simulink model "sRes_nt"  (R2018b)
settings: Solver=ode23tb  StartTime=0.0  StopTime=7  MaxStep=10e-6  RelTol=1e-4  EnableMultiTasking=on
libraries: powerlib x49
settings Model: SimulationMode=accelerator  Creator=Gong Linxiao  LastModifiedBy=vibra
settings DataIOCC: LimitDataPoints=on  SaveFormat=Array
settings OptimizationCC: LifeSpan=inf
settings DebuggingCC: SolverPrmCheckMsg=warning  SFUnexpectedBacktrackingDiag=warning  SFNoUnconditionalDefaultTransitionDiag=warning  SFExecutionAtInitializationDiag=none
settings HardwareCC: ProdBitPerPointer=32  ProdBitPerSizeT=32  ProdBitPerPtrDiffT=32  ProdLargestAtomicFloat=None  ProdIntDivRoundTo=Undefined  ProdEndianess=Unspecified  ProdWordSize=32  ProdHWDeviceType=32-bit Generic
settings ModelReferenceCC: PropagateSignalLabelsOutOfModel=off
settings SFSimCC: SimUseLocalCustomCode=off
settings RTWCC: RTWUseLocalCustomCode=off
settings CodeAppCC: StateflowObjectComments=on
settings GRTTargetCC: TargetLangStandard=C89/C90 (ANSI)  GeneratePreprocessorConditionals=Disable all
settings ConfigComp: CovMetricSettings=dw  CovHtmlReporting=on  CovSaveCumulativeToWorkspaceVar=on  CovSaveSingleToWorkspaceVar=on  CovExternalEMLEnable=off  CovSFcnEnable=off
settings SimscapeCC: SimscapeNormalizeSystem=off

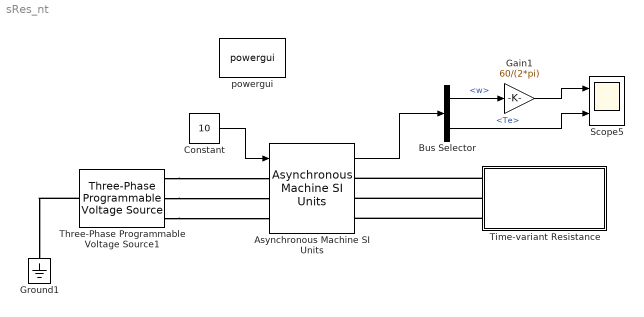
== system sRes_nt ==
  Asynchronous Machine SI Units : powerlib/Machines/Asynchronous Machine SI Units  RotorType=Wound  PresetModel="15:  5.4 HP (4KW)   400 V  50Hz 1430 RPM"  MechanicalLoad=Torque Tm  ShowDetailedParameters=on  ReferenceFrame=Stationary  Units=SI  MeasurementBus=on  NominalParameters=[4000 400 50]  Stator=[1.405 0.005839]  Rotor=[1.395 0.005839]  Cage1=[ 0.022 0.226/377]  Cage2=[ 0.022 0.226/377]  Lm=0.1722  Mechanical=[0.0131 0.002985 2]  PolePairs=2  InitialConditions=[1 0 0 0 0 0 0 0]  SimulateSaturation=off  Saturation=[14.03593122, 27.81365428, 53.79336849, 72.68890987, 97.98006896, 148.6815601, 215.7428561, 302.9841135, 420.4778367 ; 230, 322, 414, 460, 506, 552, 598, 644, 690]  LoadFlowParameters=1492000  TsPowergui=0  TsBlock=-1  IterativeModel=Trapezoidal non iterative  IterativeDiscreteModel=Trapezoidal non iterative  Pmec=0
      settings: SourceProductName=Simscape Electrical
  Bus Selector : BusSelector  OutputSignals=w,Te
  Constant : Constant  Value=10  SampleTime=Inf
  Gain1 : Gain  Gain=60/(2*pi)
  Ground1 : powerlib/Elements/Ground  LConnTagsString=a
      settings: SourceProductName=Simscape Electrical
  Scope5 : Scope  NumInputPorts=2
  Three-Phase Programmable Voltage Source1 : powerlib/Electrical Sources/Three-Phase Programmable Voltage Source  PositiveSequence="[400  0 50]"  VariationEntity=None  VariationType=Table of time-amplitude pairs  VariationTypeAlt=Step  VariationStep=20  VariationRate=30  VariationMagnitude=0.3  VariationFrequency=2  VariationTiming=[1 5]  VariationPhaseA=off  Amplitudes=[1 0.8 1.2 1.0]  TimeValues=[0 0.1 0.15 0.2]  HarmonicGeneration=off  HarmonicA=[3 0.2 -25 0]  HarmonicB=[2 0.15 35 2]  Timing="[0.05  3]"  BusType=PV  Pref=0  Qref=0  Qmin=-inf  Qmax=inf
      settings: SourceProductName=Simscape Electrical
  Time-variant Resistance : Subsystem
  powergui : powerlib/powergui  Priority=1  SimulationMode=Continuous  SampleTime=50e-6  frequency=60  Iterations=50  frequencyindice=50  Pbase=100e6  ErrMax=1e-4  UnitsV=kV  UnitsW=MW  buscounter=0  FunctionMessages=off  echomessages=off  EnableUseOfTLC=off  CurrentSourceSwitches=on  DisableSnubberDevices=off  DisableRonSwitches=off  DisableVfSwitches=off  DisplayEquations=off  SolverType=Tustin  Interpol=off  ExternalGateDelay=off  methode=off  Ts=0  x0status=steady  SPID=off  SwTol=0  HookPort=off  RestoreLinks=warning  ResistiveCurrentMeasurement=off  Frange=[0:2:500]  Ylog=off  Xlog=on  ShowGrid=off  save=off  variable=ZData  structure=0  ZoomFFT=off  StartTime=0.0  cycles=1  DisplayStyle=1  fundamental=60  FreqAxis=off  MaxFrequency=1000  frequencyindicesteady=1  RmsSteady=2  display=off
  wires:
  Constant/1 -> Asynchronous Machine SI Units/1
  Asynchronous Machine SI Units/1 -> Bus Selector/1
  Bus Selector/1 -> Gain1/1  "<w>"
  Gain1/1 -> Scope5/1
  Bus Selector/2 -> Scope5/2  "<Te>"
  connections:
  Three-Phase Programmable Voltage Source1/LConn1 -- Ground1/LConn1
  Three-Phase Programmable Voltage Source1/RConn1 -- Asynchronous Machine SI Units/LConn1
  Three-Phase Programmable Voltage Source1/RConn2 -- Asynchronous Machine SI Units/LConn2
  Three-Phase Programmable Voltage Source1/RConn3 -- Asynchronous Machine SI Units/LConn3
  Time-variant Resistance/LConn1 -- Asynchronous Machine SI Units/RConn1
  Time-variant Resistance/LConn2 -- Asynchronous Machine SI Units/RConn2
  Time-variant Resistance/LConn3 -- Asynchronous Machine SI Units/RConn3

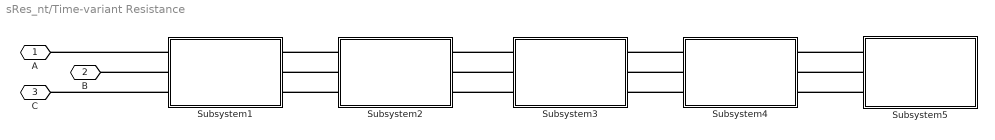
== system sRes_nt/Time-variant Resistance ==
  Subsystem1 : Subsystem
  Subsystem2 : Subsystem
  Subsystem3 : Subsystem
  Subsystem4 : Subsystem
  Subsystem5 : Subsystem
  A : PMIOPort  Side=Left
  B : PMIOPort  Port=2  Side=Left
  C : PMIOPort  Port=3  Side=Left
  connections:
  Subsystem3/LConn3 -- Subsystem2/RConn3
  Subsystem2/LConn2 -- Subsystem1/RConn2
  Subsystem3/LConn2 -- Subsystem2/RConn2
  Subsystem2/LConn3 -- Subsystem1/RConn3
  Subsystem1/LConn3 -- C/RConn1
  Subsystem4/LConn3 -- Subsystem3/RConn3
  Subsystem5/LConn2 -- Subsystem4/RConn2
  Subsystem4/LConn2 -- Subsystem3/RConn2
  Subsystem3/LConn1 -- Subsystem2/RConn1
  Subsystem4/LConn1 -- Subsystem3/RConn1
  Subsystem5/LConn1 -- Subsystem4/RConn1
  Subsystem2/LConn1 -- Subsystem1/RConn1
  Subsystem5/LConn3 -- Subsystem4/RConn3
  Subsystem1/LConn2 -- B/RConn1
  Subsystem1/LConn1 -- A/RConn1

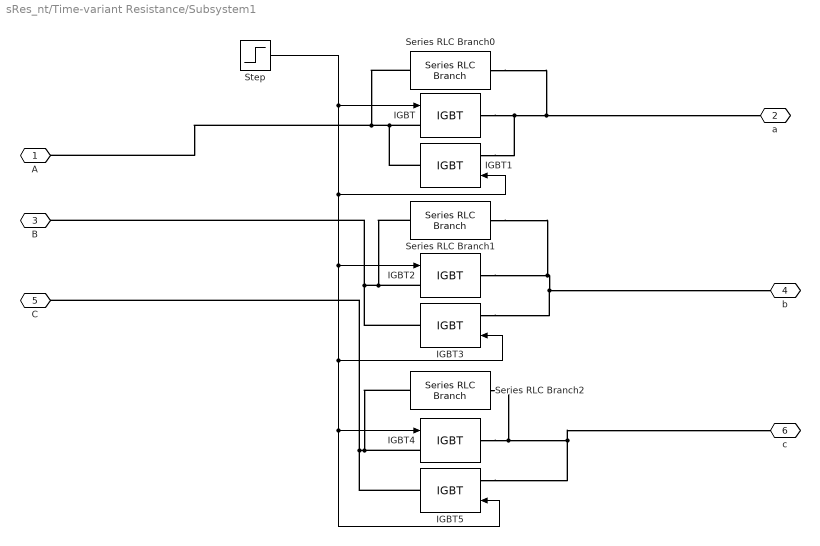
== system sRes_nt/Time-variant Resistance/Subsystem1 ==
  IGBT{,1..5} (6 alike) : powerlib/Power Electronics/IGBT  Ron=1e-5  Lon=0  Vf=0  Tf=1e-6  Tt=2e-6  IC=0  Rs=inf  Cs=inf  Measurements=off
  Series RLC Branch0 : powerlib/Elements/Series RLC Branch  LConnTagsString=__new0  RConnTagsString=__new0  BranchType=R  Resistance=1  Inductance=1e-3  SetiL0=off  InitialCurrent=0  Capacitance=1e-6  Setx0=off  InitialVoltage=0  Measurements=None
  Series RLC Branch1 : powerlib/Elements/Series RLC Branch  LConnTagsString=__new0  RConnTagsString=__new0  BranchType=R  Resistance=1  Inductance=1e-3  SetiL0=off  InitialCurrent=0  Capacitance=1e-6  Setx0=off  InitialVoltage=0  Measurements=None
  Series RLC Branch2 : powerlib/Elements/Series RLC Branch  LConnTagsString=__new0  RConnTagsString=__new0  BranchType=R  Resistance=1  Inductance=1e-3  SetiL0=off  InitialCurrent=0  Capacitance=1e-6  Setx0=off  InitialVoltage=0  Measurements=None
  Step : Step  Before=1  After=0  SampleTime=0
  A : PMIOPort  Side=Left
  a : PMIOPort  Port=2  Side=Right
  B : PMIOPort  Port=3  Side=Left
  b : PMIOPort  Port=4  Side=Right
  C : PMIOPort  Port=5  Side=Left
  c : PMIOPort  Port=6  Side=Right
  wires:
  Step/1 -> IGBT2/1, IGBT5/1, IGBT4/1, IGBT3/1, IGBT1/1, IGBT/1
  connections:
  IGBT2/RConn1 -- Series RLC Branch1/RConn1 -- b/RConn1 -- IGBT3/LConn1
  IGBT4/LConn1 -- Series RLC Branch2/LConn1 -- C/RConn1 -- IGBT5/RConn1
  IGBT4/RConn1 -- Series RLC Branch2/RConn1 -- c/RConn1 -- IGBT5/LConn1
  IGBT/LConn1 -- IGBT1/RConn1 -- A/RConn1 -- Series RLC Branch0/LConn1
  IGBT2/LConn1 -- Series RLC Branch1/LConn1 -- B/RConn1 -- IGBT3/RConn1
  IGBT/RConn1 -- IGBT1/LConn1 -- a/RConn1 -- Series RLC Branch0/RConn1

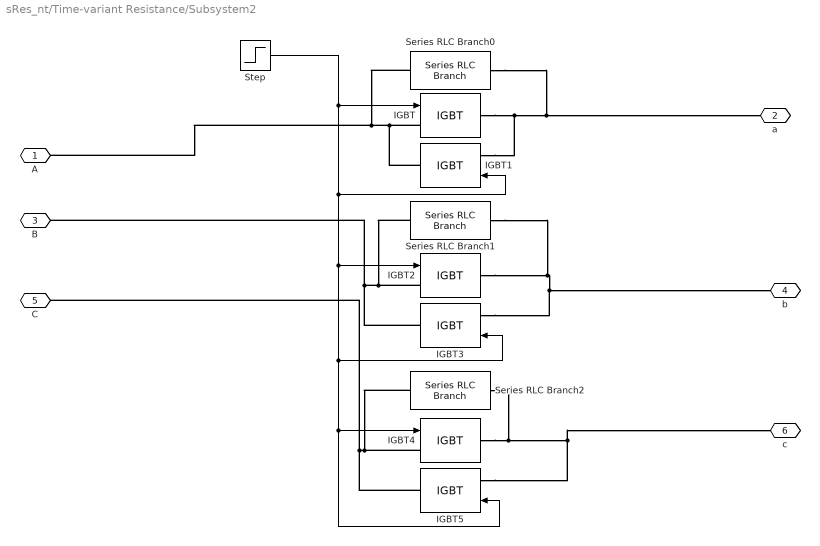
== system sRes_nt/Time-variant Resistance/Subsystem2 ==
  IGBT{,1..5} (6 alike) : powerlib/Power Electronics/IGBT  Ron=1e-5  Lon=0  Vf=0  Tf=1e-6  Tt=2e-6  IC=0  Rs=inf  Cs=inf  Measurements=off
  Series RLC Branch0 : powerlib/Elements/Series RLC Branch  LConnTagsString=__new0  RConnTagsString=__new0  BranchType=R  Resistance=1  Inductance=1e-3  SetiL0=off  InitialCurrent=0  Capacitance=1e-6  Setx0=off  InitialVoltage=0  Measurements=None
  Series RLC Branch1 : powerlib/Elements/Series RLC Branch  LConnTagsString=__new0  RConnTagsString=__new0  BranchType=R  Resistance=1  Inductance=1e-3  SetiL0=off  InitialCurrent=0  Capacitance=1e-6  Setx0=off  InitialVoltage=0  Measurements=None
  Series RLC Branch2 : powerlib/Elements/Series RLC Branch  LConnTagsString=__new0  RConnTagsString=__new0  BranchType=R  Resistance=1  Inductance=1e-3  SetiL0=off  InitialCurrent=0  Capacitance=1e-6  Setx0=off  InitialVoltage=0  Measurements=None
  Step : Step  Time=2  Before=1  After=0  SampleTime=0
  A : PMIOPort  Side=Left
  a : PMIOPort  Port=2  Side=Right
  B : PMIOPort  Port=3  Side=Left
  b : PMIOPort  Port=4  Side=Right
  C : PMIOPort  Port=5  Side=Left
  c : PMIOPort  Port=6  Side=Right
  wires:
  Step/1 -> IGBT2/1, IGBT5/1, IGBT4/1, IGBT3/1, IGBT1/1, IGBT/1
  connections:
  Series RLC Branch1/RConn1 -- IGBT2/RConn1 -- IGBT3/LConn1 -- b/RConn1
  Series RLC Branch2/LConn1 -- IGBT4/LConn1 -- IGBT5/RConn1 -- C/RConn1
  Series RLC Branch2/RConn1 -- IGBT4/RConn1 -- IGBT5/LConn1 -- c/RConn1
  Series RLC Branch0/LConn1 -- IGBT1/RConn1 -- IGBT/LConn1 -- A/RConn1
  Series RLC Branch1/LConn1 -- IGBT2/LConn1 -- IGBT3/RConn1 -- B/RConn1
  Series RLC Branch0/RConn1 -- IGBT1/LConn1 -- IGBT/RConn1 -- a/RConn1

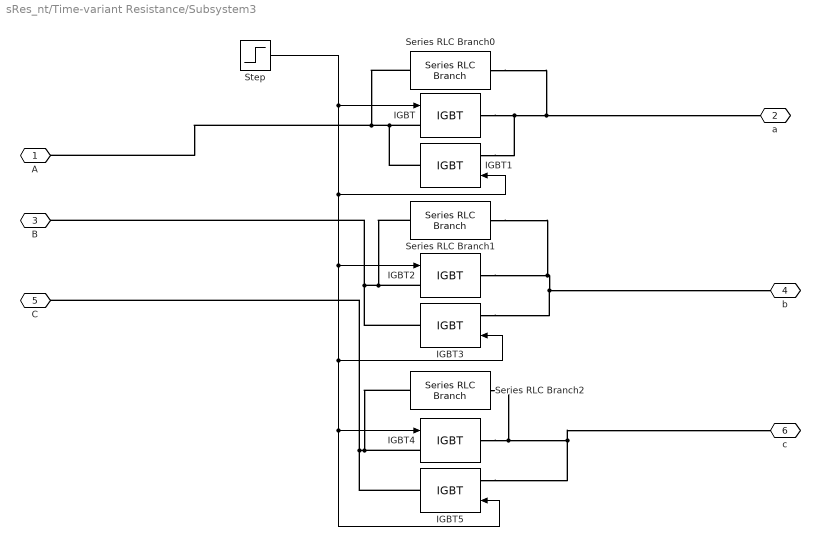
== system sRes_nt/Time-variant Resistance/Subsystem3 ==
  IGBT{,1..5} (6 alike) : powerlib/Power Electronics/IGBT  Ron=1e-5  Lon=0  Vf=0  Tf=1e-6  Tt=2e-6  IC=0  Rs=inf  Cs=inf  Measurements=off
  Series RLC Branch0 : powerlib/Elements/Series RLC Branch  LConnTagsString=__new0  RConnTagsString=__new0  BranchType=R  Resistance=1  Inductance=1e-3  SetiL0=off  InitialCurrent=0  Capacitance=1e-6  Setx0=off  InitialVoltage=0  Measurements=None
  Series RLC Branch1 : powerlib/Elements/Series RLC Branch  LConnTagsString=__new0  RConnTagsString=__new0  BranchType=R  Resistance=1  Inductance=1e-3  SetiL0=off  InitialCurrent=0  Capacitance=1e-6  Setx0=off  InitialVoltage=0  Measurements=None
  Series RLC Branch2 : powerlib/Elements/Series RLC Branch  LConnTagsString=__new0  RConnTagsString=__new0  BranchType=R  Resistance=1  Inductance=1e-3  SetiL0=off  InitialCurrent=0  Capacitance=1e-6  Setx0=off  InitialVoltage=0  Measurements=None
  Step : Step  Time=3  Before=1  After=0  SampleTime=0
  A : PMIOPort  Side=Left
  a : PMIOPort  Port=2  Side=Right
  B : PMIOPort  Port=3  Side=Left
  b : PMIOPort  Port=4  Side=Right
  C : PMIOPort  Port=5  Side=Left
  c : PMIOPort  Port=6  Side=Right
  wires:
  Step/1 -> IGBT2/1, IGBT5/1, IGBT4/1, IGBT3/1, IGBT1/1, IGBT/1
  connections:
  Series RLC Branch1/RConn1 -- IGBT2/RConn1 -- IGBT3/LConn1 -- b/RConn1
  Series RLC Branch2/LConn1 -- IGBT4/LConn1 -- IGBT5/RConn1 -- C/RConn1
  Series RLC Branch2/RConn1 -- IGBT4/RConn1 -- IGBT5/LConn1 -- c/RConn1
  Series RLC Branch0/LConn1 -- IGBT1/RConn1 -- IGBT/LConn1 -- A/RConn1
  Series RLC Branch1/LConn1 -- IGBT2/LConn1 -- IGBT3/RConn1 -- B/RConn1
  Series RLC Branch0/RConn1 -- IGBT1/LConn1 -- IGBT/RConn1 -- a/RConn1

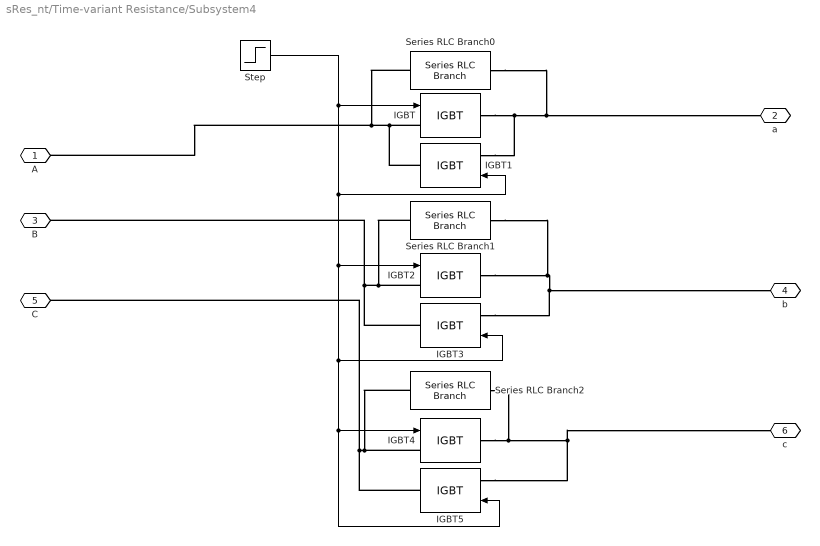
== system sRes_nt/Time-variant Resistance/Subsystem4 ==
  IGBT{,1..5} (6 alike) : powerlib/Power Electronics/IGBT  Ron=1e-5  Lon=0  Vf=0  Tf=1e-6  Tt=2e-6  IC=0  Rs=inf  Cs=inf  Measurements=off
  Series RLC Branch0 : powerlib/Elements/Series RLC Branch  LConnTagsString=__new0  RConnTagsString=__new0  BranchType=R  Resistance=1  Inductance=1e-3  SetiL0=off  InitialCurrent=0  Capacitance=1e-6  Setx0=off  InitialVoltage=0  Measurements=None
  Series RLC Branch1 : powerlib/Elements/Series RLC Branch  LConnTagsString=__new0  RConnTagsString=__new0  BranchType=R  Resistance=1  Inductance=1e-3  SetiL0=off  InitialCurrent=0  Capacitance=1e-6  Setx0=off  InitialVoltage=0  Measurements=None
  Series RLC Branch2 : powerlib/Elements/Series RLC Branch  LConnTagsString=__new0  RConnTagsString=__new0  BranchType=R  Resistance=1  Inductance=1e-3  SetiL0=off  InitialCurrent=0  Capacitance=1e-6  Setx0=off  InitialVoltage=0  Measurements=None
  Step : Step  Time=4  Before=1  After=0  SampleTime=0
  A : PMIOPort  Side=Left
  a : PMIOPort  Port=2  Side=Right
  B : PMIOPort  Port=3  Side=Left
  b : PMIOPort  Port=4  Side=Right
  C : PMIOPort  Port=5  Side=Left
  c : PMIOPort  Port=6  Side=Right
  wires:
  Step/1 -> IGBT2/1, IGBT5/1, IGBT4/1, IGBT3/1, IGBT1/1, IGBT/1
  connections:
  Series RLC Branch1/RConn1 -- IGBT2/RConn1 -- IGBT3/LConn1 -- b/RConn1
  Series RLC Branch2/LConn1 -- IGBT4/LConn1 -- IGBT5/RConn1 -- C/RConn1
  Series RLC Branch2/RConn1 -- IGBT4/RConn1 -- IGBT5/LConn1 -- c/RConn1
  Series RLC Branch0/LConn1 -- IGBT1/RConn1 -- IGBT/LConn1 -- A/RConn1
  Series RLC Branch1/LConn1 -- IGBT2/LConn1 -- IGBT3/RConn1 -- B/RConn1
  Series RLC Branch0/RConn1 -- IGBT1/LConn1 -- IGBT/RConn1 -- a/RConn1

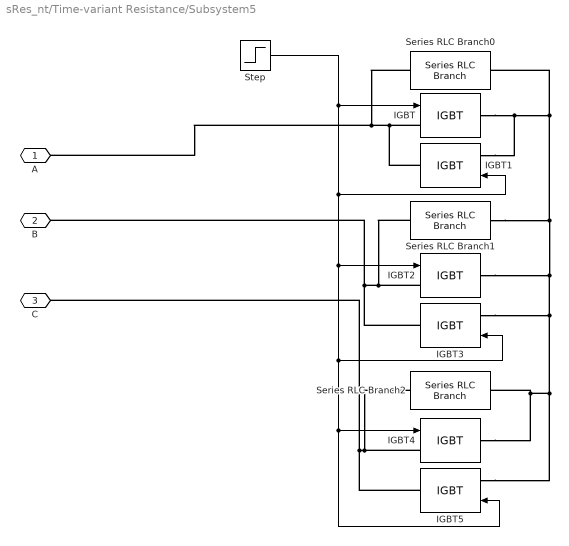
== system sRes_nt/Time-variant Resistance/Subsystem5 ==
  IGBT{,1..5} (6 alike) : powerlib/Power Electronics/IGBT  Ron=1e-5  Lon=0  Vf=0  Tf=1e-6  Tt=2e-6  IC=0  Rs=inf  Cs=inf  Measurements=off
  Series RLC Branch0 : powerlib/Elements/Series RLC Branch  LConnTagsString=__new0  RConnTagsString=__new0  BranchType=R  Resistance=1  Inductance=1e-3  SetiL0=off  InitialCurrent=0  Capacitance=1e-6  Setx0=off  InitialVoltage=0  Measurements=None
  Series RLC Branch1 : powerlib/Elements/Series RLC Branch  LConnTagsString=__new0  RConnTagsString=__new0  BranchType=R  Resistance=1  Inductance=1e-3  SetiL0=off  InitialCurrent=0  Capacitance=1e-6  Setx0=off  InitialVoltage=0  Measurements=None
  Series RLC Branch2 : powerlib/Elements/Series RLC Branch  LConnTagsString=__new0  RConnTagsString=__new0  BranchType=R  Resistance=1  Inductance=1e-3  SetiL0=off  InitialCurrent=0  Capacitance=1e-6  Setx0=off  InitialVoltage=0  Measurements=None
  Step : Step  Time=5  Before=1  After=0  SampleTime=0
  A : PMIOPort  Side=Left
  B : PMIOPort  Port=2  Side=Left
  C : PMIOPort  Port=3  Side=Left
  wires:
  Step/1 -> IGBT2/1, IGBT5/1, IGBT4/1, IGBT3/1, IGBT1/1, IGBT/1
  connections:
  Series RLC Branch2/LConn1 -- IGBT4/LConn1 -- IGBT5/RConn1 -- C/RConn1
  Series RLC Branch0/LConn1 -- IGBT1/RConn1 -- IGBT/LConn1 -- A/RConn1
  Series RLC Branch1/LConn1 -- IGBT2/LConn1 -- IGBT3/RConn1 -- B/RConn1
  Series RLC Branch1/RConn1 -- IGBT2/RConn1 -- Series RLC Branch2/RConn1 -- IGBT4/RConn1 -- IGBT5/LConn1 -- IGBT3/LConn1 -- IGBT1/LConn1 -- IGBT/RConn1 -- Series RLC Branch0/RConn1
